simulink model "idsm_second_order"  (R2023a)
settings: Solver=FixedStepDiscrete  StartTime=0.0  StopTime=65  FixedStep=1  RelTol=1e-3
values from neighbouring files (symbols this model uses):
  vin = vin_sweep(i)    [run_idsm_second_order.m]
undefined symbols (not defined in the file or in its folder): DiscIntNeverNeededParam
settings Model: Creator=bmurm  LastModifiedBy=bmurm

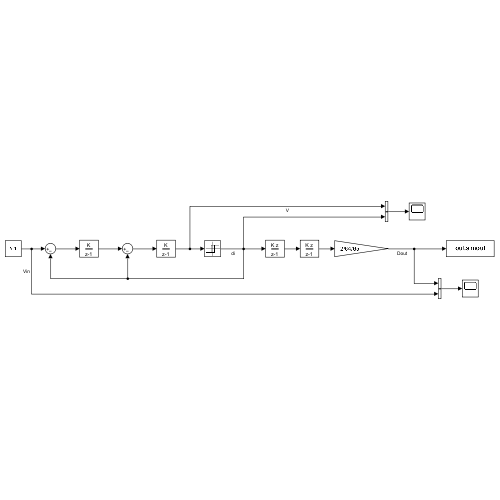
[thumbnail: Simulink's stored preview of the top-level diagram]
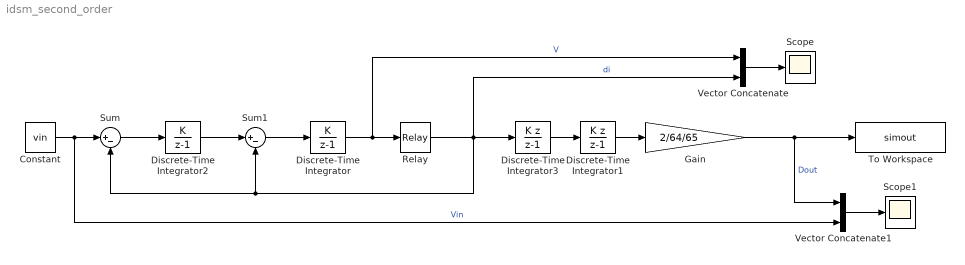
== system idsm_second_order ==
  Constant : Constant  Value=vin
  Discrete-Time Integrator : DiscreteIntegrator  IntegratorMethod=Accumulation: Forward Euler  gainval=0.5  SampleTime=-1  ICPrevOutput=DiscIntNeverNeededParam  ICPrevScaledInput=DiscIntNeverNeededParam
  Discrete-Time Integrator1 : DiscreteIntegrator  IntegratorMethod=Accumulation: Backward Euler  SampleTime=-1  ICPrevOutput=DiscIntNeverNeededParam  ICPrevScaledInput=DiscIntNeverNeededParam
  Discrete-Time Integrator2 : DiscreteIntegrator  IntegratorMethod=Accumulation: Forward Euler  gainval=0.5  SampleTime=-1  ICPrevOutput=DiscIntNeverNeededParam  ICPrevScaledInput=DiscIntNeverNeededParam
  Discrete-Time Integrator3 : DiscreteIntegrator  IntegratorMethod=Accumulation: Backward Euler  SampleTime=-1  ICPrevOutput=DiscIntNeverNeededParam  ICPrevScaledInput=DiscIntNeverNeededParam
  Gain : Gain  Gain=2/64/65
  Relay : Relay
  Scope : Scope
  Scope1 : Scope
  Sum : Sum  Inputs=|+-
  Sum1 : Sum  Inputs=|+-
  To Workspace : ToWorkspace  VariableName=simout  SaveFormat=Structure With Time  SampleTime=-1
  Vector Concatenate : Concatenate
  Vector Concatenate1 : Concatenate
  wires:
  Sum/1 -> Discrete-Time Integrator2/1
  Discrete-Time Integrator/1 -> Vector Concatenate/1, Relay/1  "V"
  Relay/1 -> Discrete-Time Integrator3/1, Vector Concatenate/2, Sum1/2, Sum/2  "di"
  Vector Concatenate/1 -> Scope/1
  Constant/1 -> Vector Concatenate1/2, Sum/1  "Vin"
  Vector Concatenate1/1 -> Scope1/1
  Discrete-Time Integrator1/1 -> Gain/1
  Gain/1 -> To Workspace/1, Vector Concatenate1/1  "Dout"
  Sum1/1 -> Discrete-Time Integrator/1
  Discrete-Time Integrator2/1 -> Sum1/1
  Discrete-Time Integrator3/1 -> Discrete-Time Integrator1/1
